simulink model "autosar_tpc_composition"  (R2022b)
settings: Solver=FixedStepDiscrete  StartTime=0.0  StopTime=10.0  RelTol=1e-3  EnableMultiTasking=on
undefined symbols (not defined in the file or in its folder): D1, P
libraries: autosarlibdem x1, autosarlibnvm x1
settings Model: Creator=The MathWorks, Inc.  LastModifiedBy=tsen
settings SolverCC: AlgebraicLoopSolver=TrustRegion  AutoInsertRateTranBlk=on  InsertRTBMode=Never (minimum delay)  MaxZcPerStep=1
settings OptimizationCC: DefaultParameterBehavior=Inlined  EnhancedBackFolding=on  PassReuseOutputArgsAs=Individual arguments  ZeroExternalMemoryAtStartup=off  ZeroInternalMemoryAtStartup=off  OptimizeBlockOrder=speed  DifferentSizesBufferReuse=on  OptimizationCustomize=off  EfficientTunableParamExpr=on
settings DebuggingCC: MultiTaskDSMMsg=none  MultiTaskRateTransMsg=warning  ParameterTunabilityLossMsg=error  UnconnectedLineMsg=warning  SFMachineParentedDataDiag=warning
settings ModelReferenceCC: EnableRefExpFcnMdlSchedulingChecks=on
settings SFSimCC: MATLABDynamicMemAlloc=off
settings RTWCC: Description=AUTOSAR  SystemTargetFile=autosar.tlc  GenCodeOnly=on  TemplateMakefile=ert_default_tmf  GenerateReport=on  IncludeHyperlinkInReport=on  LaunchReport=on  GenerateTraceInfo=on  GenerateTraceReport=on  GenerateTraceReportSl=on  GenerateTraceReportSf=on  GenerateTraceReportEml=on  DLArmComputeVersion=19.05
settings CodeAppCC: ForceParamTrailComments=on  IgnoreCustomStorageClasses=off  OperatorAnnotations=on  SimulinkDataObjDesc=on  SFDataObjDesc=on  InsertBlockDesc=on
settings STFCustomTargetCC: TargetLangStandard=C99 (ISO)  MultiwordLength=256  ParMdlRefBuildCompliant=on  CompOptLevelCompliant=on  IncludeMdlTerminateFcn=off  CombineOutputUpdateFcns=on  SuppressErrorStatus=on  ERTCustomFileBanners=on  SupportNonFinite=off  SupportComplex=off  SupportContinuousTime=off  SupportNonInlinedSFcns=off  RemoveResetFunc=on  MATLABClassNameForMDSCustomization=Simulink.SoftwareTarget.ERTCustomization  AutosarCompliant=on  UseToolchainInfoCompliant=on  LookupTableObjectStructAxisOrder=2,1,3,4,...  LUTObjectStructOrderEvenSpacing=Size,Table,Breakpoints  SystemTargetFile=autosar.tlc
settings ERTTargetCC: TargetLangStandard=C99 (ISO)  ConcurrentExecutionCompliant=off  IncludeMdlTerminateFcn=off  SuppressErrorStatus=on  SupportNonFinite=off  SupportComplex=off  ModelStepFunctionPrototypeControlCompliant=off  CPPClassGenCompliant=off  AutosarCompliant=on  LookupTableObjectStructAxisOrder=2,1,3,4,...  LUTObjectStructOrderEvenSpacing=Size,Table,Breakpoints  InlinedParameterPlacement=NonHierarchical  ERTCustomFileTemplate=example_file_process.tlc

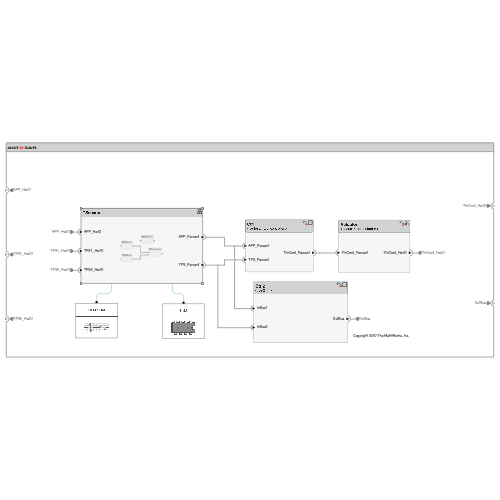
[thumbnail: Simulink's stored preview of the top-level diagram]
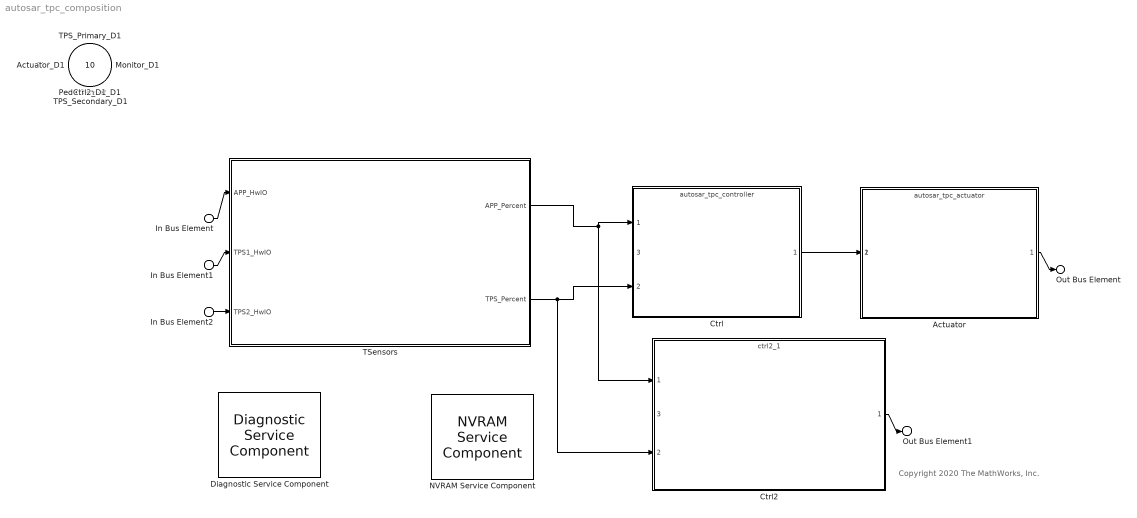
== system autosar_tpc_composition ==
  note: Copyright 2020 The MathWorks, Inc.
  In Bus Element : Inport  PortName=APP_HwIO
  In Bus Element1 : Inport  Port=2  PortName=TPS1_HwIO
  In Bus Element2 : Inport  Port=3  PortName=TPS2_HwIO
  PedalSensor_D1 : Inport  Priority=1  Port=4  OutputFunctionCall=on
  TPS_Primary_D1 : Inport  Priority=2  Port=5  OutputFunctionCall=on
  TPS_Secondary_D1 : Inport  Priority=3  Port=6  OutputFunctionCall=on
  Monitor_D1 : Inport  Priority=4  Port=7  OutputFunctionCall=on
  Ctrl_D1 : Inport  Priority=5  Port=8  OutputFunctionCall=on
  Actuator_D1 : Inport  Priority=6  Port=9  OutputFunctionCall=on
  Ctrl2_D1 : Inport  Priority=7  Port=10  OutputFunctionCall=on
  Actuator : ModelReference  ModelNameDialog=autosar_tpc_actuator.slx  SimulationMode=Normal  ScheduleRates=on  CachedPortDiscreteRates=[0.005]  ModelEventPortInfo=P:D1[0.005][0][0]  ModelReferenceVersion=6.0
      settings: PortSchema="{\"entries\":[{\"content\":{\"headerSize\":38,\"margin\":15,\"minimumSpacing\":25,\"sides\":[{\"content\":{\"connectorIds\":[\"In1\"]},\"type\":\"ConnectorPlacement.EquallySpacedRectSide\",\"uuid\":\"26fd7ed6-1773-482a-a7b4-c0bab0c01c6e\"},{\"content\":{\"connectorIds\":[\"Out1\"],\"side\":\"RIGHT\"},\"type\":\"ConnectorPlacement.EquallySpacedRectSide\",\"uuid\":\"76751916-8837-4aff-8479-b4617ededb25\"},{\"content\":{\"connectorIds\":[],\"side\":\"TOP\"},\"type\":\"ConnectorPlacement.EquallySpacedRectSide\",\"uuid\":\"b9915de3-15c1-4354-81f8-a4ac649be3ef\"},{\"content\":{\"connectorIds\":[\"In2\"],\"side\":\"HIDDEN\"},\"type\":\"ConnectorPlacement.EquallySpacedRectSide\",\"uuid\":\"40d65919-f4eb-4776-bf43-cf06a01516c0\"}]},\"type\":\"ConnectorPlacement.EquallySpacedConnector\",\"uuid\":\"5d928bdd-7cbf-4ffd-a89b-6f4194195412\"}],\"packageUris\":[\"http://schema.mathworks.com/mf0/Connector/R2020b\"],\"version\":\"1.0\"}"
  Ctrl : ModelReference  ModelNameDialog=autosar_tpc_controller.slx  SimulationMode=Normal  ScheduleRates=on  CachedPortDiscreteRates=[0.005]  ModelEventPortInfo=P:D1[0.005][0][0]  ModelReferenceVersion=6.0
      settings: PortSchema="{\"entries\":[{\"content\":{\"headerSize\":38,\"margin\":15,\"minimumSpacing\":25,\"sides\":[{\"content\":{\"connectorIds\":[\"In1\",\"In2\"]},\"type\":\"ConnectorPlacement.EquallySpacedRectSide\",\"uuid\":\"26fd7ed6-1773-482a-a7b4-c0bab0c01c6e\"},{\"content\":{\"connectorIds\":[\"Out1\"],\"side\":\"RIGHT\"},\"type\":\"ConnectorPlacement.EquallySpacedRectSide\",\"uuid\":\"76751916-8837-4aff-8479-b4617ededb25\"},{\"content\":{\"connectorIds\":[],\"side\":\"TOP\"},\"type\":\"ConnectorPlacement.EquallySpacedRectSide\",\"uuid\":\"b9915de3-15c1-4354-81f8-a4ac649be3ef\"},{\"content\":{\"connectorIds\":[\"In3\"],\"side\":\"HIDDEN\"},\"type\":\"ConnectorPlacement.EquallySpacedRectSide\",\"uuid\":\"7d1ff73c-edfa-4f44-bf72-30bebcb581a7\"}]},\"type\":\"ConnectorPlacement.EquallySpacedConnector\",\"uuid\":\"5d928bdd-7cbf-4ffd-a89b-6f4194195412\"}],\"packageUris\":[\"http://schema.mathworks.com/mf0/Connector/R2020b\"],\"version\":\"1.0\"}"
  Ctrl2 : ModelReference  ModelNameDialog=ctrl2_1  SimulationMode=Normal  ScheduleRates=on  CachedPortDiscreteRates=[0.2]  ModelEventPortInfo=P:D1[0.2][0][0]  CodeInterface=Top model  ModelReferenceVersion=2.7
      settings: PortSchema="{\"entries\":[{\"content\":{\"headerSize\":38,\"margin\":15,\"minimumSpacing\":25,\"sides\":[{\"content\":{\"connectorIds\":[\"In1\",\"In2\"]},\"type\":\"ConnectorPlacement.EquallySpacedRectSide\",\"uuid\":\"ef81b2f0-9e2a-47b4-9da0-52924950b8a3\"},{\"content\":{\"connectorIds\":[\"Out1\"],\"side\":\"RIGHT\"},\"type\":\"ConnectorPlacement.EquallySpacedRectSide\",\"uuid\":\"66d247a8-5b4f-49c4-b2a6-5af564e47947\"},{\"content\":{\"connectorIds\":[],\"side\":\"TOP\"},\"type\":\"ConnectorPlacement.EquallySpacedRectSide\",\"uuid\":\"825b5de4-29ca-4cb9-ab2e-7f7d8a7cd7e2\"},{\"content\":{\"connectorIds\":[\"In3\"],\"side\":\"HIDDEN\"},\"type\":\"ConnectorPlacement.EquallySpacedRectSide\",\"uuid\":\"174ea556-6342-438f-86fb-f76093d185aa\"}]},\"type\":\"ConnectorPlacement.EquallySpacedConnector\",\"uuid\":\"e6e6b96c-273e-44c5-b4f4-7a3f615bf1cf\"}],\"packageUris\":[\"http://schema.mathworks.com/mf0/Connector/R2020b\"],\"version\":\"1.0\"}"
  Diagnostic Service Component : autosarlibdem/Diagnostic Service Component  ClientPortNames={'S1StuckHigh', 'S1StuckLow', 'S2StuckHigh', 'S2StuckLow', 'TPS', 'TPS1StuckHigh', 'TPS1StuckLow', 'TPS2StuckHigh', 'TPS2StuckLow'}  ClientPortPortDefinedArguments={'1', '2', '3', '4', '5', '1', '2', '3', '4'}  MaxEventId=10  MaxFID=10  DemDebounceCounterIncrementStepSize=1  DemDebounceCounterDecrementStepSize=1  DemDebounceCounterFailedThreshold=2  DemDebounceCounterPassedThreshold=-1  InhibitionMatrix=zeros(11,'uint8')  EnableConditionIndexes=zeros(257,'uint8')  StorageConditionIndexes=zeros(257,'uint8')
  NVRAM Service Component : autosarlibnvm/NVRAM Service Component  ClientPortNames={'S1LowSetPoint', 'S2LowSetPoint'}  ClientPortPortDefinedArguments={'1', '2'}  MaxBlockId=10  NvInitValues={'0'}
  TSensors : Subsystem
      settings: PortSchema="{\"entries\":[{\"content\":{\"headerSize\":26,\"margin\":15,\"minimumSpacing\":25,\"sides\":[{\"content\":{\"connectorIds\":[\"In3\",\"In1\",\"In2\"]},\"type\":\"ConnectorPlacement.EquallySpacedRectSide\",\"uuid\":\"26fd7ed6-1773-482a-a7b4-c0bab0c01c6e\"},{\"content\":{\"connectorIds\":[\"Out1\",\"Out2\"],\"side\":\"RIGHT\"},\"type\":\"ConnectorPlacement.EquallySpacedRectSide\",\"uuid\":\"76751916-8837-4aff-8479-b4617ededb25\"},{\"content\":{\"connectorIds\":[],\"side\":\"TOP\"},\"type\":\"ConnectorPlacement.EquallySpacedRectSide\",\"uuid\":\"b9915de3-15c1-4354-81f8-a4ac649be3ef\"}]},\"type\":\"ConnectorPlacement.EquallySpacedConnector\",\"uuid\":\"5d928bdd-7cbf-4ffd-a89b-6f4194195412\"}],\"packageUris\":[\"http://schema.mathworks.com/mf0/Connector/R2020b\"],\"version\":\"1.0\"}"
  Out Bus Element : Outport  PortName=ThrCmd_HwIO
  Out Bus Element1 : Outport  Port=2  PortName=OutBus
  wires:
  Ctrl/1 -> Actuator/1
  Actuator/1 -> Out Bus Element/1
  In Bus Element/1 -> TSensors/3(APP_HwIO)
  In Bus Element1/1 -> TSensors/1(TPS1_HwIO)
  In Bus Element2/1 -> TSensors/2(TPS2_HwIO)
  TSensors/2(TPS_Percent) -> Ctrl2/2, Ctrl/2
  TSensors/1(APP_Percent) -> Ctrl2/1, Ctrl/1
  Ctrl2/1 -> Out Bus Element1/1

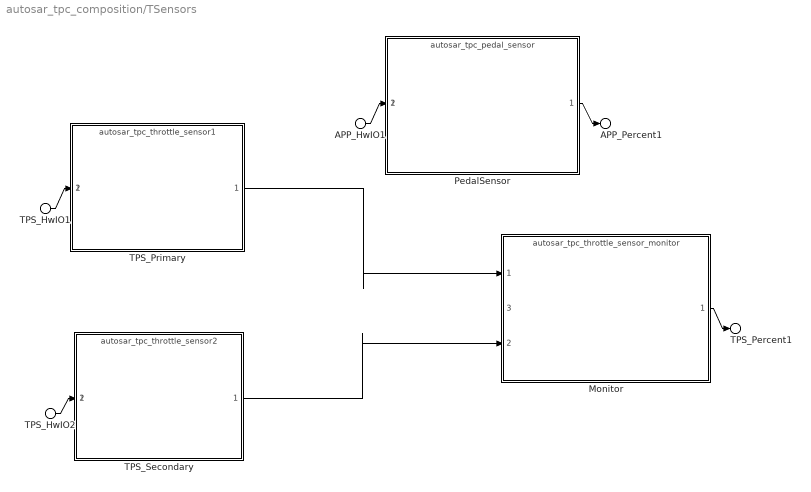
== system autosar_tpc_composition/TSensors ==
  TPS_HwIO1 : Inport  PortName=TPS1_HwIO
  TPS_HwIO2 : Inport  Port=2  PortName=TPS2_HwIO
  APP_HwIO1 : Inport  Port=3  PortName=APP_HwIO
  Monitor : ModelReference  ModelNameDialog=autosar_tpc_throttle_sensor_monitor.slx  SimulationMode=Normal  ScheduleRates=on  CachedPortDiscreteRates=[0.005]  ModelEventPortInfo=P:D1[0.005][0][0]  ModelReferenceVersion=5.1
      settings: PortSchema="{\"entries\":[{\"content\":{\"headerSize\":38,\"margin\":15,\"minimumSpacing\":25,\"sides\":[{\"content\":{\"connectorIds\":[\"In1\",\"In2\"]},\"type\":\"ConnectorPlacement.EquallySpacedRectSide\",\"uuid\":\"26fd7ed6-1773-482a-a7b4-c0bab0c01c6e\"},{\"content\":{\"connectorIds\":[\"Out1\"],\"side\":\"RIGHT\"},\"type\":\"ConnectorPlacement.EquallySpacedRectSide\",\"uuid\":\"76751916-8837-4aff-8479-b4617ededb25\"},{\"content\":{\"connectorIds\":[],\"side\":\"TOP\"},\"type\":\"ConnectorPlacement.EquallySpacedRectSide\",\"uuid\":\"b9915de3-15c1-4354-81f8-a4ac649be3ef\"},{\"content\":{\"connectorIds\":[\"In3\"],\"side\":\"HIDDEN\"},\"type\":\"ConnectorPlacement.EquallySpacedRectSide\",\"uuid\":\"302746d1-7dce-4aba-b330-892e2c60171f\"}]},\"type\":\"ConnectorPlacement.EquallySpacedConnector\",\"uuid\":\"5d928bdd-7cbf-4ffd-a89b-6f4194195412\"}],\"packageUris\":[\"http://schema.mathworks.com/mf0/Connector/R2020b\"],\"version\":\"1.0\"}"
  PedalSensor : ModelReference  ModelNameDialog=autosar_tpc_pedal_sensor.slx  SimulationMode=Normal  ScheduleRates=on  CachedPortDiscreteRates=[0.005]  ModelEventPortInfo=P:D1[0.005][0][0]  ModelReferenceVersion=5.2
      settings: PortSchema="{\"entries\":[{\"content\":{\"headerSize\":38,\"margin\":15,\"minimumSpacing\":25,\"sides\":[{\"content\":{\"connectorIds\":[\"In1\"]},\"type\":\"ConnectorPlacement.EquallySpacedRectSide\",\"uuid\":\"26fd7ed6-1773-482a-a7b4-c0bab0c01c6e\"},{\"content\":{\"connectorIds\":[\"Out1\"],\"side\":\"RIGHT\"},\"type\":\"ConnectorPlacement.EquallySpacedRectSide\",\"uuid\":\"76751916-8837-4aff-8479-b4617ededb25\"},{\"content\":{\"connectorIds\":[],\"side\":\"TOP\"},\"type\":\"ConnectorPlacement.EquallySpacedRectSide\",\"uuid\":\"b9915de3-15c1-4354-81f8-a4ac649be3ef\"},{\"content\":{\"connectorIds\":[\"In2\"],\"side\":\"HIDDEN\"},\"type\":\"ConnectorPlacement.EquallySpacedRectSide\",\"uuid\":\"32803b45-a236-4461-aef0-ac45c73929d4\"}]},\"type\":\"ConnectorPlacement.EquallySpacedConnector\",\"uuid\":\"5d928bdd-7cbf-4ffd-a89b-6f4194195412\"}],\"packageUris\":[\"http://schema.mathworks.com/mf0/Connector/R2020b\"],\"version\":\"1.0\"}"
  TPS_Primary : ModelReference  ModelNameDialog=autosar_tpc_throttle_sensor1.slx  SimulationMode=Normal  ScheduleRates=on  CachedPortDiscreteRates=[0.005]  ModelEventPortInfo=P:D1[0.005][0][0]  ModelReferenceVersion=4.1
      settings: PortSchema="{\"entries\":[{\"content\":{\"headerSize\":38,\"margin\":15,\"minimumSpacing\":25,\"sides\":[{\"content\":{\"connectorIds\":[\"In1\"]},\"type\":\"ConnectorPlacement.EquallySpacedRectSide\",\"uuid\":\"26fd7ed6-1773-482a-a7b4-c0bab0c01c6e\"},{\"content\":{\"connectorIds\":[\"Out1\"],\"side\":\"RIGHT\"},\"type\":\"ConnectorPlacement.EquallySpacedRectSide\",\"uuid\":\"76751916-8837-4aff-8479-b4617ededb25\"},{\"content\":{\"connectorIds\":[],\"side\":\"TOP\"},\"type\":\"ConnectorPlacement.EquallySpacedRectSide\",\"uuid\":\"b9915de3-15c1-4354-81f8-a4ac649be3ef\"},{\"content\":{\"connectorIds\":[\"In2\"],\"side\":\"HIDDEN\"},\"type\":\"ConnectorPlacement.EquallySpacedRectSide\",\"uuid\":\"72449d16-bda2-4078-95c4-c90e16bab07f\"}]},\"type\":\"ConnectorPlacement.EquallySpacedConnector\",\"uuid\":\"5d928bdd-7cbf-4ffd-a89b-6f4194195412\"}],\"packageUris\":[\"http://schema.mathworks.com/mf0/Connector/R2020b\"],\"version\":\"1.0\"}"
  TPS_Secondary : ModelReference  ModelNameDialog=autosar_tpc_throttle_sensor2.slx  SimulationMode=Normal  ScheduleRates=on  CachedPortDiscreteRates=[0.005]  ModelEventPortInfo=P:D1[0.005][0][0]  ModelReferenceVersion=4.1
      settings: PortSchema="{\"entries\":[{\"content\":{\"headerSize\":38,\"margin\":15,\"minimumSpacing\":25,\"sides\":[{\"content\":{\"connectorIds\":[\"In1\"]},\"type\":\"ConnectorPlacement.EquallySpacedRectSide\",\"uuid\":\"26fd7ed6-1773-482a-a7b4-c0bab0c01c6e\"},{\"content\":{\"connectorIds\":[\"Out1\"],\"side\":\"RIGHT\"},\"type\":\"ConnectorPlacement.EquallySpacedRectSide\",\"uuid\":\"76751916-8837-4aff-8479-b4617ededb25\"},{\"content\":{\"connectorIds\":[],\"side\":\"TOP\"},\"type\":\"ConnectorPlacement.EquallySpacedRectSide\",\"uuid\":\"b9915de3-15c1-4354-81f8-a4ac649be3ef\"},{\"content\":{\"connectorIds\":[\"In2\"],\"side\":\"HIDDEN\"},\"type\":\"ConnectorPlacement.EquallySpacedRectSide\",\"uuid\":\"f03159cf-3720-4778-a44c-a02363af00e8\"}]},\"type\":\"ConnectorPlacement.EquallySpacedConnector\",\"uuid\":\"5d928bdd-7cbf-4ffd-a89b-6f4194195412\"}],\"packageUris\":[\"http://schema.mathworks.com/mf0/Connector/R2020b\"],\"version\":\"1.0\"}"
  APP_Percent1 : Outport  PortName=APP_Percent
  TPS_Percent1 : Outport  Port=2  PortName=TPS_Percent
  wires:
  TPS_HwIO1/1 -> TPS_Primary/1
  TPS_HwIO2/1 -> TPS_Secondary/1
  APP_HwIO1/1 -> PedalSensor/1
  PedalSensor/1 -> APP_Percent1/1
  Monitor/1 -> TPS_Percent1/1
  TPS_Primary/1 -> Monitor/1
  TPS_Secondary/1 -> Monitor/2
